simulink model "paralines_2"  (Simulink 8.5)
settings: Solver=ode15s  SolverMode=SingleTasking  StartTime=0.0  StopTime=0.2  RelTol=1e-3  AbsTol=1e-6
libraries: powerlib x64
settings Model: Creator=Dr. Lotfifard  LastModifiedBy=PC
settings DataIOCC: LimitDataPoints=off
settings OptimizationCC: BlockReduction=off  BooleanDataType=off
settings DebuggingCC: SaveWithParameterizedLinksMsg=none  SignalResolutionControl=TryResolveAllWithWarning  MultiTaskDSMMsg=warning  MultiTaskCondExecSysMsg=none  FcnCallInpInsideContextMsg=UseLocalSettings  StrictBusMsg=None
settings HardwareCC: TargetUnknown=on

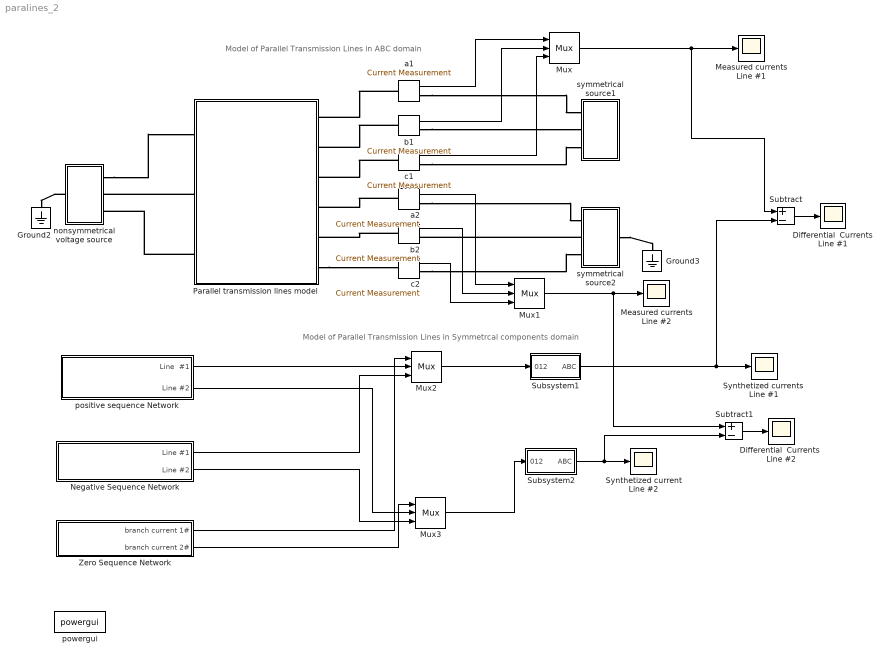
== system paralines_2 ==
  note: Model of Parallel Transmission Lines in ABC domain
  note: Model of Parallel Transmission Lines in Symmetrcal components domain
  " Synthetized current Line #2" : Scope
      settings: TickLabels=on  TimeRange=0.1  YMin=-20  YMax=20
  " Synthetized currents  Line #1" : Scope
      settings: TickLabels=on  TimeRange=0.1  YMin=-30  YMax=30  SaveName=ScopeData2
  Differential  Currents Line #1 : Scope
      settings: TickLabels=on  TimeRange=0.07000000000000001  YMin=-10  YMax=10  SaveName=ScopeData3
  Differential  Currents  Line #2 : Scope
      settings: TickLabels=on  TimeRange=0.07000000000000001  YMin=-10  YMax=10  SaveName=ScopeData4
  Ground2 : powerlib/Elements/Ground  LConnTagsString=a
  Ground3 : powerlib/Elements/Ground  LConnTagsString=a
  Measured currents Line #1 : Scope
      settings: TickLabels=on  TimeRange=0.1  YMin=-30  YMax=30  SaveName=ScopeData5
  Measured currents Line #2 : Scope
      settings: TickLabels=on  TimeRange=0.1  YMin=-20  YMax=20
  Mux{,1..3} (4 alike) : Mux  Inputs=3
  Negative Sequence Network : Subsystem
  Parallel transmission lines model : Subsystem
  Subsystem1 : Subsystem
  Subsystem2 : Subsystem
  Subtract : Sum  Inputs=+-  SaturateOnIntegerOverflow=on  InputSameDT=on  OutDataTypeStr=Inherit: Same as first input
  Subtract1 : Sum  Inputs=+-  SaturateOnIntegerOverflow=on  InputSameDT=on  OutDataTypeStr=Inherit: Same as first input
  Zero Sequence Network : Subsystem
  a1 : powerlib/Measurements/Current Measurement  PhasorSimulation=off  OutputType=Complex  PSBequivalent=0
  a2 : powerlib/Measurements/Current Measurement  PhasorSimulation=off  OutputType=Complex  PSBequivalent=0
  b1 : powerlib/Measurements/Current Measurement  PhasorSimulation=off  OutputType=Complex  PSBequivalent=0
  b2 : powerlib/Measurements/Current Measurement  PhasorSimulation=off  OutputType=Complex  PSBequivalent=0
  c1 : powerlib/Measurements/Current Measurement  PhasorSimulation=off  OutputType=Complex  PSBequivalent=0
  c2 : powerlib/Measurements/Current Measurement  PhasorSimulation=off  OutputType=Complex  PSBequivalent=0
  nonsymmetrical voltage source : Subsystem
  positive sequence Network : Subsystem
  powergui : powerlib/powergui  SimulationMode=Continuous  SolverType=Tustin/Backward Euler (TBE)  SampleTime=0  frequency=60  SPID=off  DisableSnubberDevices=off  DisableRonSwitches=off  DisableVfSwitches=off  SwTol=0  DisplayEquations=off  Interpol=off  methode=off  Ts=0  FunctionMessages=off  echomessages=off  HookPort=off  EnableUseOfTLC=off  x0status=blocks  frequencyindice=60  Pbase=100e6  ErrMax=1e-4  Iterations=50  UnitsV=kV  UnitsW=MW  buscounter=0  RestoreLinks=warning  ResistiveCurrentMeasurement=off  Frange=[0:2:500]  Ylog=off  Xlog=on  ShowGrid=off  save=off  variable=ZData  structure=0  ZoomFFT=on  StartTime=0.0  cycles=1  DisplayStyle=1  fundamental=60  FreqAxis=off  MaxFrequency=1000  frequencyindicesteady=1  RmsSteady=1  display=off
  symmetrical source1 : Subsystem
  symmetrical source2 : Subsystem
  wires:
  Mux3/1 -> Subsystem2/1(012)
  positive sequence Network/1(Line  #1) -> Mux2/2
  Negative Sequence Network/1(Line #1) -> Mux2/3
  Mux2/1 -> Subsystem1/1(012)
  positive sequence Network/2(Line #2) -> Mux3/2
  a1/1 -> Mux/1
  c1/1 -> Mux/3
  b1/1 -> Mux/2
  a2/1 -> Mux1/1
  b2/1 -> Mux1/2
  c2/1 -> Mux1/3
  Subtract/1 -> Differential  Currents Line #1/1
  Mux/1 -> Measured currents Line #1/1, Subtract/1
  Subsystem1/1(ABC) -> " Synthetized currents  Line #1"/1, Subtract/2
  Subtract1/1 -> Differential  Currents  Line #2/1
  Mux1/1 -> Measured currents Line #2/1, Subtract1/1
  Subsystem2/1(ABC) -> " Synthetized current Line #2"/1, Subtract1/2
  Negative Sequence Network/2(Line #2) -> Mux3/3
  Zero Sequence Network/1(branch current 1#) -> Mux2/1
  Zero Sequence Network/2(branch current 2#) -> Mux3/1
  connections:
  nonsymmetrical voltage source/LConn1 -- Ground2/LConn1
  a2/LConn1 -- Parallel transmission lines model/RConn4
  Parallel transmission lines model/LConn2 -- nonsymmetrical voltage source/RConn2
  Parallel transmission lines model/LConn3 -- nonsymmetrical voltage source/RConn3
  nonsymmetrical voltage source/RConn1 -- Parallel transmission lines model/LConn1
  b2/LConn1 -- Parallel transmission lines model/RConn5
  a1/LConn1 -- Parallel transmission lines model/RConn1
  b1/LConn1 -- Parallel transmission lines model/RConn2
  a2/RConn1 -- symmetrical source2/RConn1
  c1/RConn1 -- symmetrical source1/RConn3
  c1/LConn1 -- Parallel transmission lines model/RConn3
  symmetrical source2/LConn1 -- Ground3/LConn1
  symmetrical source2/RConn2 -- b2/RConn1
  a1/RConn1 -- symmetrical source1/RConn1
  c2/RConn1 -- symmetrical source2/RConn3
  b1/RConn1 -- symmetrical source1/RConn2
  Parallel transmission lines model/RConn6 -- c2/LConn1

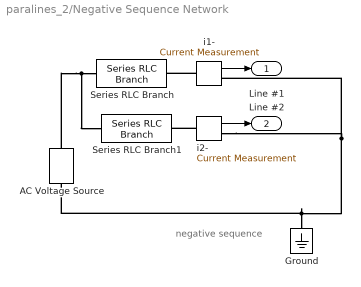
== system paralines_2/Negative Sequence Network ==
  note: negative sequence
  AC Voltage Source : powerlib/Electrical Sources/AC Voltage Source  Amplitude=10*(1.732-1)/3  Phase=30  Frequency=60  SampleTime=0  Measurements=None
  Ground : powerlib/Elements/Ground  LConnTagsString=a
  Series RLC Branch : powerlib/Elements/Series RLC Branch  LConnTagsString=__new0  RConnTagsString=__new0  BranchType=RL  Resistance=(1e-3)  Inductance=(0.5-0.1)/(2*pi*60)  SetiL0=off  InitialCurrent=0  Capacitance=1e-6  Setx0=off  InitialVoltage=0  Measurements=None
  Series RLC Branch1 : powerlib/Elements/Series RLC Branch  LConnTagsString=__new0  RConnTagsString=__new0  BranchType=RL  Resistance=(1e-3)  Inductance=(0.5-0.1)/(2*pi*60)  SetiL0=off  InitialCurrent=0  Capacitance=1e-6  Setx0=off  InitialVoltage=0  Measurements=None
  i1- : powerlib/Measurements/Current Measurement  PhasorSimulation=off  OutputType=Complex  PSBequivalent=0
  i2- : powerlib/Measurements/Current Measurement  PhasorSimulation=off  OutputType=Complex  PSBequivalent=0
  Line #1 : Outport  InitialOutput=0
  Line #2 : Outport  Port=2  InitialOutput=0
  wires:
  i1-/1 -> Line #1/1
  i2-/1 -> Line #2/1
  connections:
  Series RLC Branch/LConn1 -- Series RLC Branch1/LConn1 -- AC Voltage Source/RConn1
  Ground/LConn1 -- i1-/RConn1 -- i2-/RConn1 -- AC Voltage Source/LConn1
  i1-/LConn1 -- Series RLC Branch/RConn1
  i2-/LConn1 -- Series RLC Branch1/RConn1

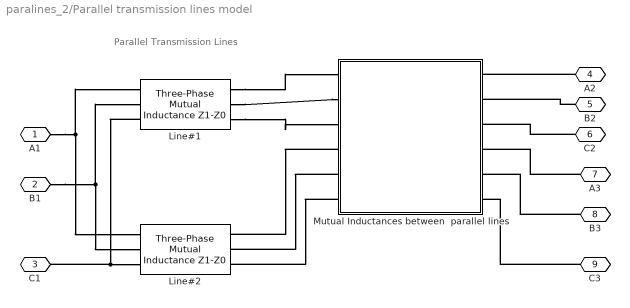
== system paralines_2/Parallel transmission lines model ==
  note: Parallel Transmission Lines
  Line#1 : powerlib/Elements/Three-Phase Mutual Inductance Z1-Z0  LConnTagsString=a|b|c  RConnTagsString=A|B|C  PositiveSequence="[1e-3  0.4/(2*pi*60) ]"  ZeroSequence="[1e-3  0.7/(2*pi*60) ]"
  Line#2 : powerlib/Elements/Three-Phase Mutual Inductance Z1-Z0  LConnTagsString=a|b|c  RConnTagsString=A|B|C  PositiveSequence="[1e-3  0.4/(2*pi*60) ]"  ZeroSequence="[1e-3  0.7/(2*pi*60) ]"
  Mutual Inductances between  parallel lines : Subsystem  mask{Lm=0.01}
      mask prompts: Lm "Mutual inductance between phases in different lines (Ohm)"
      mask Display: disp('Mutual \nCoupling\n model\n for the\n parallel lines')
  A1 : PMIOPort  Port=1  Side=Left
  B1 : PMIOPort  Port=2  Side=Left
  C1 : PMIOPort  Port=3  Side=Left
  A2 : PMIOPort  Port=4  Side=Right
  B2 : PMIOPort  Port=5  Side=Right
  C2 : PMIOPort  Port=6  Side=Right
  A3 : PMIOPort  Port=7  Side=Right
  B3 : PMIOPort  Port=8  Side=Right
  C3 : PMIOPort  Port=9  Side=Right
  connections:
  A1/RConn1 -- Line#1/LConn1 -- Line#2/LConn1
  B1/RConn1 -- Line#1/LConn2 -- Line#2/LConn2
  Line#1/LConn3 -- C1/RConn1 -- Line#2/LConn3
  Line#1/RConn1 -- Mutual Inductances between  parallel lines/LConn1
  Line#1/RConn2 -- Mutual Inductances between  parallel lines/LConn2
  Line#1/RConn3 -- Mutual Inductances between  parallel lines/LConn3
  Mutual Inductances between  parallel lines/LConn4 -- Line#2/RConn1
  Mutual Inductances between  parallel lines/LConn5 -- Line#2/RConn2
  Mutual Inductances between  parallel lines/LConn6 -- Line#2/RConn3
  A2/RConn1 -- Mutual Inductances between  parallel lines/RConn1
  B2/RConn1 -- Mutual Inductances between  parallel lines/RConn2
  C2/RConn1 -- Mutual Inductances between  parallel lines/RConn3
  A3/RConn1 -- Mutual Inductances between  parallel lines/RConn4
  B3/RConn1 -- Mutual Inductances between  parallel lines/RConn5
  C3/RConn1 -- Mutual Inductances between  parallel lines/RConn6

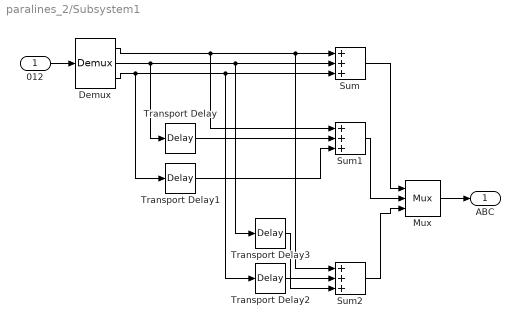
== system paralines_2/Subsystem1 ==
  012 : Inport
  Demux : Demux  Outputs=3
  Mux : Mux  Inputs=3
  Sum : Sum  Inputs=+++  SaturateOnIntegerOverflow=on  InputSameDT=on  OutDataTypeStr=Inherit: Same as first input
  Sum1 : Sum  Inputs=+++  SaturateOnIntegerOverflow=on  InputSameDT=on  OutDataTypeStr=Inherit: Same as first input
  Sum2 : Sum  Inputs=+++  SaturateOnIntegerOverflow=on  InputSameDT=on  OutDataTypeStr=Inherit: Same as first input
  Transport Delay : TransportDelay  DelayTime=1/(3*60)
  Transport Delay1 : TransportDelay  DelayTime=2/(3*60)
  Transport Delay2 : TransportDelay  DelayTime=1/(3*60)
  Transport Delay3 : TransportDelay  DelayTime=2/(3*60)
  ABC : Outport  InitialOutput=0
  wires:
  012/1 -> Demux/1
  Sum1/1 -> Mux/2
  Sum/1 -> Mux/1
  Mux/1 -> ABC/1
  Sum2/1 -> Mux/3
  Demux/2 -> Transport Delay/1, Sum/2, Transport Delay3/1
  Demux/3 -> Transport Delay1/1, Sum/3, Transport Delay2/1
  Demux/1 -> Sum1/1, Sum/1, Sum2/1
  Transport Delay/1 -> Sum1/2
  Transport Delay1/1 -> Sum1/3
  Transport Delay2/1 -> Sum2/3
  Transport Delay3/1 -> Sum2/2

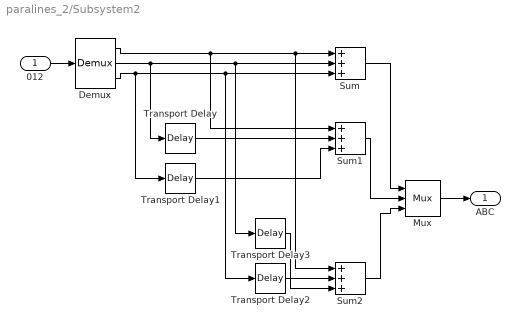
== system paralines_2/Subsystem2 ==
  012 : Inport
  Demux : Demux  Outputs=3
  Mux : Mux  Inputs=3
  Sum : Sum  Inputs=+++  SaturateOnIntegerOverflow=on  InputSameDT=on  OutDataTypeStr=Inherit: Same as first input
  Sum1 : Sum  Inputs=+++  SaturateOnIntegerOverflow=on  InputSameDT=on  OutDataTypeStr=Inherit: Same as first input
  Sum2 : Sum  Inputs=+++  SaturateOnIntegerOverflow=on  InputSameDT=on  OutDataTypeStr=Inherit: Same as first input
  Transport Delay : TransportDelay  DelayTime=1/(3*60)
  Transport Delay1 : TransportDelay  DelayTime=2/(3*60)
  Transport Delay2 : TransportDelay  DelayTime=1/(3*60)
  Transport Delay3 : TransportDelay  DelayTime=2/(3*60)
  ABC : Outport  InitialOutput=0
  wires:
  012/1 -> Demux/1
  Sum1/1 -> Mux/2
  Sum/1 -> Mux/1
  Mux/1 -> ABC/1
  Sum2/1 -> Mux/3
  Demux/2 -> Transport Delay/1, Sum/2, Transport Delay3/1
  Demux/3 -> Transport Delay1/1, Sum/3, Transport Delay2/1
  Demux/1 -> Sum1/1, Sum/1, Sum2/1
  Transport Delay/1 -> Sum1/2
  Transport Delay1/1 -> Sum1/3
  Transport Delay2/1 -> Sum2/3
  Transport Delay3/1 -> Sum2/2

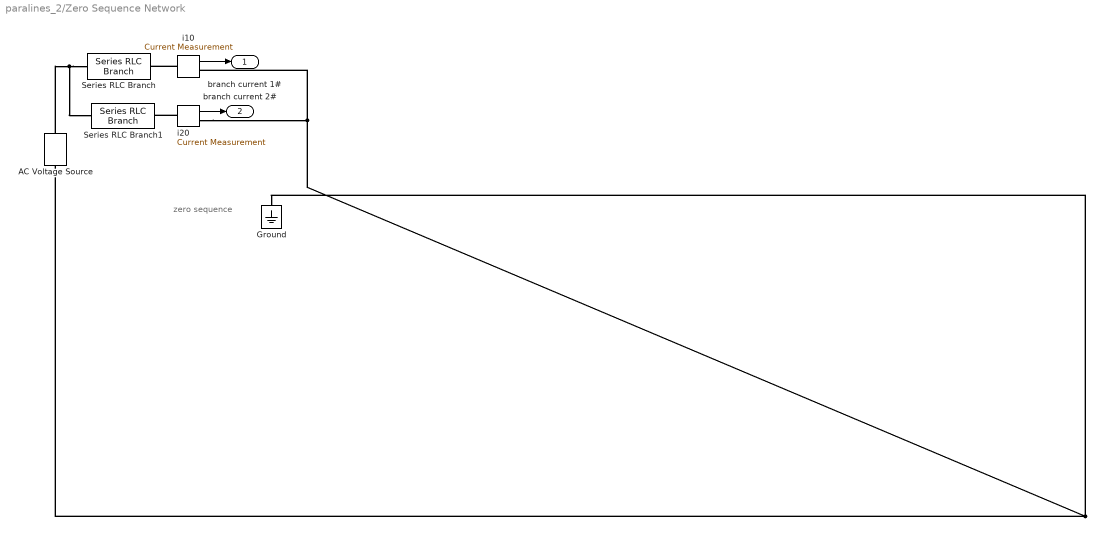
== system paralines_2/Zero Sequence Network ==
  note: zero sequence
  AC Voltage Source : powerlib/Electrical Sources/AC Voltage Source  Amplitude=10/3  Phase=90  Frequency=60  SampleTime=0  Measurements=None
  Ground : powerlib/Elements/Ground  LConnTagsString=a
  Series RLC Branch : powerlib/Elements/Series RLC Branch  LConnTagsString=__new0  RConnTagsString=__new0  BranchType=RL  Resistance=(1e-3)  Inductance=(0.5-0.1)/(2*pi*60)  SetiL0=off  InitialCurrent=0  Capacitance=1e-6  Setx0=off  InitialVoltage=0  Measurements=None
  Series RLC Branch1 : powerlib/Elements/Series RLC Branch  LConnTagsString=__new0  RConnTagsString=__new0  BranchType=RL  Resistance=(1e-3)  Inductance=(0.5-0.1)/(2*pi*60)  SetiL0=off  InitialCurrent=0  Capacitance=1e-6  Setx0=off  InitialVoltage=0  Measurements=None
  i10 : powerlib/Measurements/Current Measurement  PhasorSimulation=off  OutputType=Complex  PSBequivalent=0
  i20 : powerlib/Measurements/Current Measurement  PhasorSimulation=off  OutputType=Complex  PSBequivalent=0
  branch current 1# : Outport  InitialOutput=0
  branch current 2# : Outport  Port=2  InitialOutput=0
  wires:
  i10/1 -> branch current 1#/1
  i20/1 -> branch current 2#/1
  connections:
  Series RLC Branch/LConn1 -- Series RLC Branch1/LConn1 -- AC Voltage Source/RConn1
  i10/RConn1 -- i20/RConn1 -- AC Voltage Source/LConn1 -- Ground/LConn1
  i10/LConn1 -- Series RLC Branch/RConn1
  i20/LConn1 -- Series RLC Branch1/RConn1

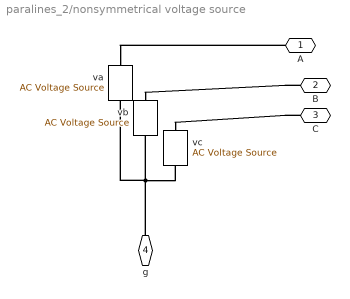
== system paralines_2/nonsymmetrical voltage source ==
  va : powerlib/Electrical Sources/AC Voltage Source  Amplitude=10  Phase=0  Frequency=60  SampleTime=0  Measurements=None
  vb : powerlib/Electrical Sources/AC Voltage Source  Amplitude=10  Phase=180  Frequency=60  SampleTime=0  Measurements=None
  vc : powerlib/Electrical Sources/AC Voltage Source  Amplitude=10  Phase=90  Frequency=60  SampleTime=0  Measurements=None
  A : PMIOPort  Port=1  Side=Right
  B : PMIOPort  Port=2  Side=Right
  C : PMIOPort  Port=3  Side=Right
  g : PMIOPort  Port=4  Side=Left
  connections:
  g/RConn1 -- vb/LConn1 -- vc/LConn1 -- va/LConn1
  A/RConn1 -- va/RConn1
  B/RConn1 -- vb/RConn1
  C/RConn1 -- vc/RConn1

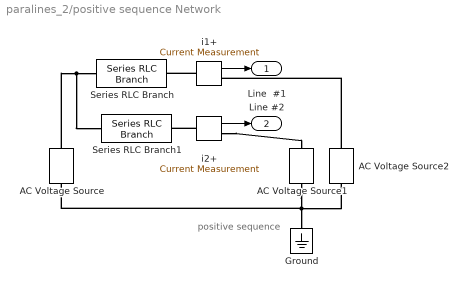
== system paralines_2/positive sequence Network ==
  note: positive sequence
  AC Voltage Source : powerlib/Electrical Sources/AC Voltage Source  Amplitude=10*(1+1.732)/3  Phase=-30  Frequency=60  SampleTime=0  Measurements=None
  AC Voltage Source1 : powerlib/Electrical Sources/AC Voltage Source  Amplitude=8  Phase=-20  Frequency=60  SampleTime=0  Measurements=None
  AC Voltage Source2 : powerlib/Electrical Sources/AC Voltage Source  Amplitude=8  Phase=20  Frequency=60  SampleTime=0  Measurements=None
  Ground : powerlib/Elements/Ground  LConnTagsString=a
  Series RLC Branch : powerlib/Elements/Series RLC Branch  LConnTagsString=__new0  RConnTagsString=__new0  BranchType=RL  Resistance=(1e-3)  Inductance=(0.5-0.1)/(2*pi*60)  SetiL0=off  InitialCurrent=0  Capacitance=1e-6  Setx0=off  InitialVoltage=0  Measurements=None
  Series RLC Branch1 : powerlib/Elements/Series RLC Branch  LConnTagsString=__new0  RConnTagsString=__new0  BranchType=RL  Resistance=(1e-3)  Inductance=(0.5-0.1)/(2*pi*60)  SetiL0=off  InitialCurrent=0  Capacitance=1e-6  Setx0=off  InitialVoltage=0  Measurements=None
  i1+ : powerlib/Measurements/Current Measurement  PhasorSimulation=off  OutputType=Complex  PSBequivalent=0
  i2+ : powerlib/Measurements/Current Measurement  PhasorSimulation=off  OutputType=Complex  PSBequivalent=0
  Line  #1 : Outport  InitialOutput=0
  Line #2 : Outport  Port=2  InitialOutput=0
  wires:
  i1+/1 -> Line  #1/1
  i2+/1 -> Line #2/1
  connections:
  i1+/LConn1 -- Series RLC Branch/RConn1
  i2+/LConn1 -- Series RLC Branch1/RConn1
  AC Voltage Source/RConn1 -- Series RLC Branch/LConn1 -- Series RLC Branch1/LConn1
  i2+/RConn1 -- AC Voltage Source1/RConn1
  AC Voltage Source2/RConn1 -- i1+/RConn1
  AC Voltage Source1/LConn1 -- AC Voltage Source/LConn1 -- AC Voltage Source2/LConn1 -- Ground/LConn1

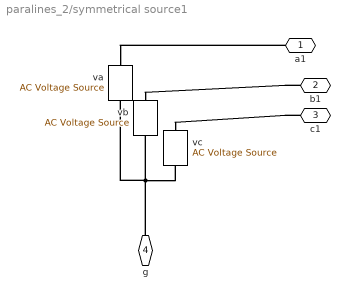
== system paralines_2/symmetrical source1 ==
  va : powerlib/Electrical Sources/AC Voltage Source  Amplitude=8  Phase=20  Frequency=60  SampleTime=0  Measurements=None
  vb : powerlib/Electrical Sources/AC Voltage Source  Amplitude=8  Phase=-100  Frequency=60  SampleTime=0  Measurements=None
  vc : powerlib/Electrical Sources/AC Voltage Source  Amplitude=8  Phase=140  Frequency=60  SampleTime=0  Measurements=None
  a1 : PMIOPort  Port=1  Side=Right
  b1 : PMIOPort  Port=2  Side=Right
  c1 : PMIOPort  Port=3  Side=Right
  g : PMIOPort  Port=4  Side=Left
  connections:
  g/RConn1 -- vb/LConn1 -- vc/LConn1 -- va/LConn1
  a1/RConn1 -- va/RConn1
  b1/RConn1 -- vb/RConn1
  c1/RConn1 -- vc/RConn1

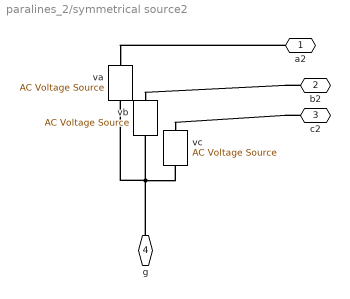
== system paralines_2/symmetrical source2 ==
  va : powerlib/Electrical Sources/AC Voltage Source  Amplitude=8  Phase=-20  Frequency=60  SampleTime=0  Measurements=None
  vb : powerlib/Electrical Sources/AC Voltage Source  Amplitude=8  Phase=-140  Frequency=60  SampleTime=0  Measurements=None
  vc : powerlib/Electrical Sources/AC Voltage Source  Amplitude=8  Phase=100  Frequency=60  SampleTime=0  Measurements=None
  a2 : PMIOPort  Port=1  Side=Right
  b2 : PMIOPort  Port=2  Side=Right
  c2 : PMIOPort  Port=3  Side=Right
  g : PMIOPort  Port=4  Side=Left
  connections:
  g/RConn1 -- vb/LConn1 -- vc/LConn1 -- va/LConn1
  a2/RConn1 -- va/RConn1
  b2/RConn1 -- vb/RConn1
  c2/RConn1 -- vc/RConn1

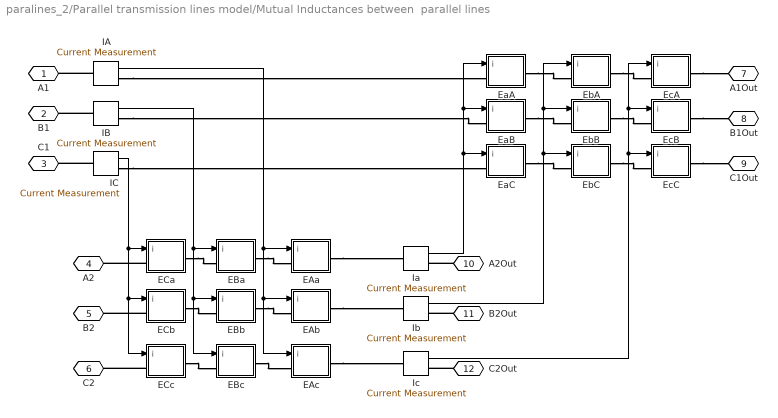
== system paralines_2/Parallel transmission lines model/Mutual Inductances between  parallel lines ==
  " EBb" : Subsystem
  " ECc" : Subsystem
  " EaA" : Subsystem
  " EaB" : Subsystem
  " EbB" : Subsystem
  " EbC" : Subsystem
  EAa : Subsystem
  EAb : Subsystem
  EAc : Subsystem
  EBa : Subsystem
  EBc : Subsystem
  "ECa " : Subsystem
  ECb : Subsystem
  EaC : Subsystem
  EbA : Subsystem
  EcA : Subsystem
  EcB : Subsystem
  EcC : Subsystem
  IA : powerlib/Measurements/Current Measurement  PhasorSimulation=off  OutputType=Complex  PSBequivalent=0
  IB : powerlib/Measurements/Current Measurement  PhasorSimulation=off  OutputType=Complex  PSBequivalent=0
  IC : powerlib/Measurements/Current Measurement  PhasorSimulation=off  OutputType=Complex  PSBequivalent=0
  Ia : powerlib/Measurements/Current Measurement  PhasorSimulation=off  OutputType=Complex  PSBequivalent=0
  Ib : powerlib/Measurements/Current Measurement  PhasorSimulation=off  OutputType=Complex  PSBequivalent=0
  Ic : powerlib/Measurements/Current Measurement  PhasorSimulation=off  OutputType=Complex  PSBequivalent=0
  A1 : PMIOPort  Port=1  Side=Left
  B1 : PMIOPort  Port=2  Side=Left
  C1 : PMIOPort  Port=3  Side=Left
  A2 : PMIOPort  Port=4  Side=Left
  B2 : PMIOPort  Port=5  Side=Left
  C2 : PMIOPort  Port=6  Side=Left
  A1Out : PMIOPort  Port=7  Side=Right
  B1Out : PMIOPort  Port=8  Side=Right
  C1Out : PMIOPort  Port=9  Side=Right
  A2Out : PMIOPort  Port=10  Side=Right
  B2Out : PMIOPort  Port=11  Side=Right
  C2Out : PMIOPort  Port=12  Side=Right
  wires:
  Ib/1 -> EbA/1(" i"), " EbB"/1(" i"), " EbC"/1(" i")
  Ic/1 -> EcA/1(" i"), EcB/1(" i"), EcC/1(" i")
  Ia/1 -> " EaA"/1(" i"), " EaB"/1(" i"), EaC/1(" i")
  IB/1 -> EBc/1(" i"), " EBb"/1(" i"), EBa/1(" i")
  IA/1 -> EAc/1(" i"), EAb/1(" i"), EAa/1(" i")
  IC/1 -> "ECa "/1(" i"), " ECc"/1(" i"), ECb/1(" i")
  connections:
  IA/LConn1 -- A1/RConn1
  IB/LConn1 -- B1/RConn1
  IC/LConn1 -- C1/RConn1
  A2Out/RConn1 -- Ia/RConn1
  B2Out/RConn1 -- Ib/RConn1
  C2Out/RConn1 -- Ic/RConn1
  EBa/RConn1 -- EAa/LConn1
  "ECa "/RConn1 -- EBa/LConn1
  " EBb"/RConn1 -- EAb/LConn1
  EBc/RConn1 -- EAc/LConn1
  " ECc"/RConn1 -- EBc/LConn1
  ECb/RConn1 -- " EBb"/LConn1
  EaC/RConn1 -- " EbC"/LConn1
  " EaB"/RConn1 -- " EbB"/LConn1
  " EaA"/RConn1 -- EbA/LConn1
  EbA/RConn1 -- EcA/LConn1
  " EbB"/RConn1 -- EcB/LConn1
  " EbC"/RConn1 -- EcC/LConn1
  EcA/RConn1 -- A1Out/RConn1
  EcB/RConn1 -- B1Out/RConn1
  EcC/RConn1 -- C1Out/RConn1
  EAa/RConn1 -- Ia/LConn1
  EAb/RConn1 -- Ib/LConn1
  EAc/RConn1 -- Ic/LConn1
  "ECa "/LConn1 -- A2/RConn1
  ECb/LConn1 -- B2/RConn1
  " ECc"/LConn1 -- C2/RConn1
  IA/RConn1 -- " EaA"/LConn1
  IB/RConn1 -- " EaB"/LConn1
  IC/RConn1 -- EaC/LConn1

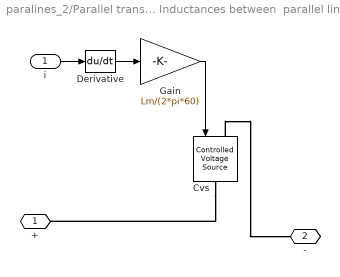
== system paralines_2/Parallel transmission lines model/Mutual Inductances between  parallel lines/ EBb ==
  " i" : Inport
  Cvs : powerlib/Electrical Sources/Controlled Voltage Source  Tag=PoWeRsYsTeMbLoCk  Initialize=on  Source_Type=AC  Amplitude=0  Phase=0  Frequency=0  Measurements=None
  Derivative : Derivative
  Gain : Gain  Gain=Lm/(2*pi*60)  SaturateOnIntegerOverflow=on  OutDataTypeStr=Inherit: Same as input  ParamDataTypeStr=Inherit: Same as input
  + : PMIOPort  Port=1  Side=Left
  - : PMIOPort  Port=2  Side=Right
  wires:
  Derivative/1 -> Gain/1
  Gain/1 -> Cvs/1
  " i"/1 -> Derivative/1
  connections:
  Cvs/LConn1 -- -/RConn1
  Cvs/RConn1 -- +/RConn1

== system paralines_2/Parallel transmission lines model/Mutual Inductances between  parallel lines/ ECc ==
  " i" : Inport
  Cvs : powerlib/Electrical Sources/Controlled Voltage Source  Tag=PoWeRsYsTeMbLoCk  Initialize=on  Source_Type=AC  Amplitude=0  Phase=0  Frequency=0  Measurements=None
  Derivative : Derivative
  Gain : Gain  Gain=Lm/(2*pi*60)  SaturateOnIntegerOverflow=on  OutDataTypeStr=Inherit: Same as input  ParamDataTypeStr=Inherit: Same as input
  + : PMIOPort  Port=1  Side=Left
  - : PMIOPort  Port=2  Side=Right
  wires:
  Derivative/1 -> Gain/1
  Gain/1 -> Cvs/1
  " i"/1 -> Derivative/1
  connections:
  Cvs/LConn1 -- -/RConn1
  Cvs/RConn1 -- +/RConn1

== system paralines_2/Parallel transmission lines model/Mutual Inductances between  parallel lines/ EaA ==
  " i" : Inport
  Cvs : powerlib/Electrical Sources/Controlled Voltage Source  Tag=PoWeRsYsTeMbLoCk  Initialize=on  Source_Type=AC  Amplitude=0  Phase=0  Frequency=0  Measurements=None
  Derivative : Derivative
  Gain : Gain  Gain=Lm/(2*pi*60)  SaturateOnIntegerOverflow=on  OutDataTypeStr=Inherit: Same as input  ParamDataTypeStr=Inherit: Same as input
  + : PMIOPort  Port=1  Side=Left
  - : PMIOPort  Port=2  Side=Right
  wires:
  Derivative/1 -> Gain/1
  Gain/1 -> Cvs/1
  " i"/1 -> Derivative/1
  connections:
  Cvs/LConn1 -- -/RConn1
  Cvs/RConn1 -- +/RConn1

== system paralines_2/Parallel transmission lines model/Mutual Inductances between  parallel lines/ EaB ==
  " i" : Inport
  Cvs : powerlib/Electrical Sources/Controlled Voltage Source  Tag=PoWeRsYsTeMbLoCk  Initialize=on  Source_Type=AC  Amplitude=0  Phase=0  Frequency=0  Measurements=None
  Derivative : Derivative
  Gain : Gain  Gain=Lm/(2*pi*60)  SaturateOnIntegerOverflow=on  OutDataTypeStr=Inherit: Same as input  ParamDataTypeStr=Inherit: Same as input
  + : PMIOPort  Port=1  Side=Left
  - : PMIOPort  Port=2  Side=Right
  wires:
  Derivative/1 -> Gain/1
  Gain/1 -> Cvs/1
  " i"/1 -> Derivative/1
  connections:
  Cvs/LConn1 -- -/RConn1
  Cvs/RConn1 -- +/RConn1

== system paralines_2/Parallel transmission lines model/Mutual Inductances between  parallel lines/ EbB ==
  " i" : Inport
  Cvs : powerlib/Electrical Sources/Controlled Voltage Source  Tag=PoWeRsYsTeMbLoCk  Initialize=on  Source_Type=AC  Amplitude=0  Phase=0  Frequency=0  Measurements=None
  Derivative : Derivative
  Gain : Gain  Gain=Lm/(2*pi*60)  SaturateOnIntegerOverflow=on  OutDataTypeStr=Inherit: Same as input  ParamDataTypeStr=Inherit: Same as input
  + : PMIOPort  Port=1  Side=Left
  - : PMIOPort  Port=2  Side=Right
  wires:
  Derivative/1 -> Gain/1
  Gain/1 -> Cvs/1
  " i"/1 -> Derivative/1
  connections:
  Cvs/LConn1 -- -/RConn1
  Cvs/RConn1 -- +/RConn1

== system paralines_2/Parallel transmission lines model/Mutual Inductances between  parallel lines/ EbC ==
  " i" : Inport
  Cvs : powerlib/Electrical Sources/Controlled Voltage Source  Tag=PoWeRsYsTeMbLoCk  Initialize=on  Source_Type=AC  Amplitude=0  Phase=0  Frequency=0  Measurements=None
  Derivative : Derivative
  Gain : Gain  Gain=Lm/(2*pi*60)  SaturateOnIntegerOverflow=on  OutDataTypeStr=Inherit: Same as input  ParamDataTypeStr=Inherit: Same as input
  + : PMIOPort  Port=1  Side=Left
  - : PMIOPort  Port=2  Side=Right
  wires:
  Derivative/1 -> Gain/1
  Gain/1 -> Cvs/1
  " i"/1 -> Derivative/1
  connections:
  Cvs/LConn1 -- -/RConn1
  Cvs/RConn1 -- +/RConn1

== system paralines_2/Parallel transmission lines model/Mutual Inductances between  parallel lines/EAa ==
  " i" : Inport
  Cvs : powerlib/Electrical Sources/Controlled Voltage Source  Tag=PoWeRsYsTeMbLoCk  Initialize=on  Source_Type=AC  Amplitude=0  Phase=0  Frequency=0  Measurements=None
  Derivative : Derivative
  Gain : Gain  Gain=Lm/(2*pi*60)  SaturateOnIntegerOverflow=on  OutDataTypeStr=Inherit: Same as input  ParamDataTypeStr=Inherit: Same as input
  + : PMIOPort  Port=1  Side=Left
  - : PMIOPort  Port=2  Side=Right
  wires:
  Derivative/1 -> Gain/1
  Gain/1 -> Cvs/1
  " i"/1 -> Derivative/1
  connections:
  Cvs/RConn1 -- +/RConn1
  Cvs/LConn1 -- -/RConn1

== system paralines_2/Parallel transmission lines model/Mutual Inductances between  parallel lines/EAb ==
  " i" : Inport
  Cvs : powerlib/Electrical Sources/Controlled Voltage Source  Tag=PoWeRsYsTeMbLoCk  Initialize=on  Source_Type=AC  Amplitude=0  Phase=0  Frequency=0  Measurements=None
  Derivative : Derivative
  Gain : Gain  Gain=Lm/(2*pi*60)  SaturateOnIntegerOverflow=on  OutDataTypeStr=Inherit: Same as input  ParamDataTypeStr=Inherit: Same as input
  + : PMIOPort  Port=1  Side=Left
  - : PMIOPort  Port=2  Side=Right
  wires:
  Derivative/1 -> Gain/1
  Gain/1 -> Cvs/1
  " i"/1 -> Derivative/1
  connections:
  Cvs/LConn1 -- -/RConn1
  Cvs/RConn1 -- +/RConn1

== system paralines_2/Parallel transmission lines model/Mutual Inductances between  parallel lines/EAc ==
  " i" : Inport
  Cvs : powerlib/Electrical Sources/Controlled Voltage Source  Tag=PoWeRsYsTeMbLoCk  Initialize=on  Source_Type=AC  Amplitude=0  Phase=0  Frequency=0  Measurements=None
  Derivative : Derivative
  Gain : Gain  Gain=Lm/(2*pi*60)  SaturateOnIntegerOverflow=on  OutDataTypeStr=Inherit: Same as input  ParamDataTypeStr=Inherit: Same as input
  + : PMIOPort  Port=1  Side=Left
  - : PMIOPort  Port=2  Side=Right
  wires:
  Derivative/1 -> Gain/1
  Gain/1 -> Cvs/1
  " i"/1 -> Derivative/1
  connections:
  Cvs/LConn1 -- -/RConn1
  Cvs/RConn1 -- +/RConn1

== system paralines_2/Parallel transmission lines model/Mutual Inductances between  parallel lines/EBa ==
  " i" : Inport
  Cvs : powerlib/Electrical Sources/Controlled Voltage Source  Tag=PoWeRsYsTeMbLoCk  Initialize=on  Source_Type=AC  Amplitude=0  Phase=0  Frequency=0  Measurements=None
  Derivative : Derivative
  Gain : Gain  Gain=Lm/(2*pi*60)  SaturateOnIntegerOverflow=on  OutDataTypeStr=Inherit: Same as input  ParamDataTypeStr=Inherit: Same as input
  + : PMIOPort  Port=1  Side=Left
  - : PMIOPort  Port=2  Side=Right
  wires:
  Derivative/1 -> Gain/1
  Gain/1 -> Cvs/1
  " i"/1 -> Derivative/1
  connections:
  Cvs/RConn1 -- +/RConn1
  Cvs/LConn1 -- -/RConn1

== system paralines_2/Parallel transmission lines model/Mutual Inductances between  parallel lines/EBc ==
  " i" : Inport
  Cvs : powerlib/Electrical Sources/Controlled Voltage Source  Tag=PoWeRsYsTeMbLoCk  Initialize=on  Source_Type=AC  Amplitude=0  Phase=0  Frequency=0  Measurements=None
  Derivative : Derivative
  Gain : Gain  Gain=Lm/(2*pi*60)  SaturateOnIntegerOverflow=on  OutDataTypeStr=Inherit: Same as input  ParamDataTypeStr=Inherit: Same as input
  + : PMIOPort  Port=1  Side=Left
  - : PMIOPort  Port=2  Side=Right
  wires:
  Derivative/1 -> Gain/1
  Gain/1 -> Cvs/1
  " i"/1 -> Derivative/1
  connections:
  Cvs/LConn1 -- -/RConn1
  Cvs/RConn1 -- +/RConn1

== system paralines_2/Parallel transmission lines model/Mutual Inductances between  parallel lines/ECa  ==
  " i" : Inport
  Cvs : powerlib/Electrical Sources/Controlled Voltage Source  Tag=PoWeRsYsTeMbLoCk  Initialize=on  Source_Type=AC  Amplitude=0  Phase=0  Frequency=0  Measurements=None
  Derivative : Derivative
  Gain : Gain  Gain=Lm/(2*pi*60)  SaturateOnIntegerOverflow=on  OutDataTypeStr=Inherit: Same as input  ParamDataTypeStr=Inherit: Same as input
  + : PMIOPort  Port=1  Side=Left
  - : PMIOPort  Port=2  Side=Right
  wires:
  Derivative/1 -> Gain/1
  Gain/1 -> Cvs/1
  " i"/1 -> Derivative/1
  connections:
  Cvs/RConn1 -- +/RConn1
  Cvs/LConn1 -- -/RConn1

== system paralines_2/Parallel transmission lines model/Mutual Inductances between  parallel lines/ECb ==
  " i" : Inport
  Cvs : powerlib/Electrical Sources/Controlled Voltage Source  Tag=PoWeRsYsTeMbLoCk  Initialize=on  Source_Type=AC  Amplitude=0  Phase=0  Frequency=0  Measurements=None
  Derivative : Derivative
  Gain : Gain  Gain=Lm/(2*pi*60)  SaturateOnIntegerOverflow=on  OutDataTypeStr=Inherit: Same as input  ParamDataTypeStr=Inherit: Same as input
  + : PMIOPort  Port=1  Side=Left
  - : PMIOPort  Port=2  Side=Right
  wires:
  Derivative/1 -> Gain/1
  Gain/1 -> Cvs/1
  " i"/1 -> Derivative/1
  connections:
  Cvs/LConn1 -- -/RConn1
  Cvs/RConn1 -- +/RConn1

== system paralines_2/Parallel transmission lines model/Mutual Inductances between  parallel lines/EaC ==
  " i" : Inport
  Cvs : powerlib/Electrical Sources/Controlled Voltage Source  Tag=PoWeRsYsTeMbLoCk  Initialize=on  Source_Type=AC  Amplitude=0  Phase=0  Frequency=0  Measurements=None
  Derivative : Derivative
  Gain : Gain  Gain=Lm/(2*pi*60)  SaturateOnIntegerOverflow=on  OutDataTypeStr=Inherit: Same as input  ParamDataTypeStr=Inherit: Same as input
  + : PMIOPort  Port=1  Side=Left
  - : PMIOPort  Port=2  Side=Right
  wires:
  Derivative/1 -> Gain/1
  Gain/1 -> Cvs/1
  " i"/1 -> Derivative/1
  connections:
  Cvs/LConn1 -- -/RConn1
  Cvs/RConn1 -- +/RConn1

== system paralines_2/Parallel transmission lines model/Mutual Inductances between  parallel lines/EbA ==
  " i" : Inport
  Cvs : powerlib/Electrical Sources/Controlled Voltage Source  Tag=PoWeRsYsTeMbLoCk  Initialize=on  Source_Type=AC  Amplitude=0  Phase=0  Frequency=0  Measurements=None
  Derivative : Derivative
  Gain : Gain  Gain=Lm/(2*pi*60)  SaturateOnIntegerOverflow=on  OutDataTypeStr=Inherit: Same as input  ParamDataTypeStr=Inherit: Same as input
  + : PMIOPort  Port=1  Side=Left
  - : PMIOPort  Port=2  Side=Right
  wires:
  Derivative/1 -> Gain/1
  Gain/1 -> Cvs/1
  " i"/1 -> Derivative/1
  connections:
  Cvs/LConn1 -- -/RConn1
  Cvs/RConn1 -- +/RConn1

== system paralines_2/Parallel transmission lines model/Mutual Inductances between  parallel lines/EcA ==
  " i" : Inport
  Cvs : powerlib/Electrical Sources/Controlled Voltage Source  Tag=PoWeRsYsTeMbLoCk  Initialize=on  Source_Type=AC  Amplitude=0  Phase=0  Frequency=0  Measurements=None
  Derivative : Derivative
  Gain : Gain  Gain=Lm/(2*pi*60)  SaturateOnIntegerOverflow=on  OutDataTypeStr=Inherit: Same as input  ParamDataTypeStr=Inherit: Same as input
  + : PMIOPort  Port=1  Side=Left
  - : PMIOPort  Port=2  Side=Right
  wires:
  Derivative/1 -> Gain/1
  Gain/1 -> Cvs/1
  " i"/1 -> Derivative/1
  connections:
  Cvs/LConn1 -- -/RConn1
  Cvs/RConn1 -- +/RConn1

== system paralines_2/Parallel transmission lines model/Mutual Inductances between  parallel lines/EcB ==
  " i" : Inport
  Cvs : powerlib/Electrical Sources/Controlled Voltage Source  Tag=PoWeRsYsTeMbLoCk  Initialize=on  Source_Type=AC  Amplitude=0  Phase=0  Frequency=0  Measurements=None
  Derivative : Derivative
  Gain : Gain  Gain=Lm/(2*pi*60)  SaturateOnIntegerOverflow=on  OutDataTypeStr=Inherit: Same as input  ParamDataTypeStr=Inherit: Same as input
  + : PMIOPort  Port=1  Side=Left
  - : PMIOPort  Port=2  Side=Right
  wires:
  Derivative/1 -> Gain/1
  Gain/1 -> Cvs/1
  " i"/1 -> Derivative/1
  connections:
  Cvs/LConn1 -- -/RConn1
  Cvs/RConn1 -- +/RConn1

== system paralines_2/Parallel transmission lines model/Mutual Inductances between  parallel lines/EcC ==
  " i" : Inport
  Cvs : powerlib/Electrical Sources/Controlled Voltage Source  Tag=PoWeRsYsTeMbLoCk  Initialize=on  Source_Type=AC  Amplitude=0  Phase=0  Frequency=0  Measurements=None
  Derivative : Derivative
  Gain : Gain  Gain=Lm/(2*pi*60)  SaturateOnIntegerOverflow=on  OutDataTypeStr=Inherit: Same as input  ParamDataTypeStr=Inherit: Same as input
  + : PMIOPort  Port=1  Side=Left
  - : PMIOPort  Port=2  Side=Right
  wires:
  Derivative/1 -> Gain/1
  Gain/1 -> Cvs/1
  " i"/1 -> Derivative/1
  connections:
  Cvs/LConn1 -- -/RConn1
  Cvs/RConn1 -- +/RConn1
